simulink model "Control_hibrido"  (R2018a)
settings: Solver=FixedStepAuto  StartTime=0.0  StopTime=20  FixedStep=1e-3  RelTol=1e-3
PreLoadFcn:
  | ej_3_init;
InitFcn:
  | ej_3_init;
StartFcn:
  | hold on;
  | patch([2 0 0 2],[0 2 2 0], [-2 -2 1 1],'g' );
undefined symbols (not defined in the file or in its folder): cfg
libraries: simulink x4, roblocks x2
CloseFcn:
  | hold off;
settings Model: Creator=Guido L  LastModifiedBy=Guido L

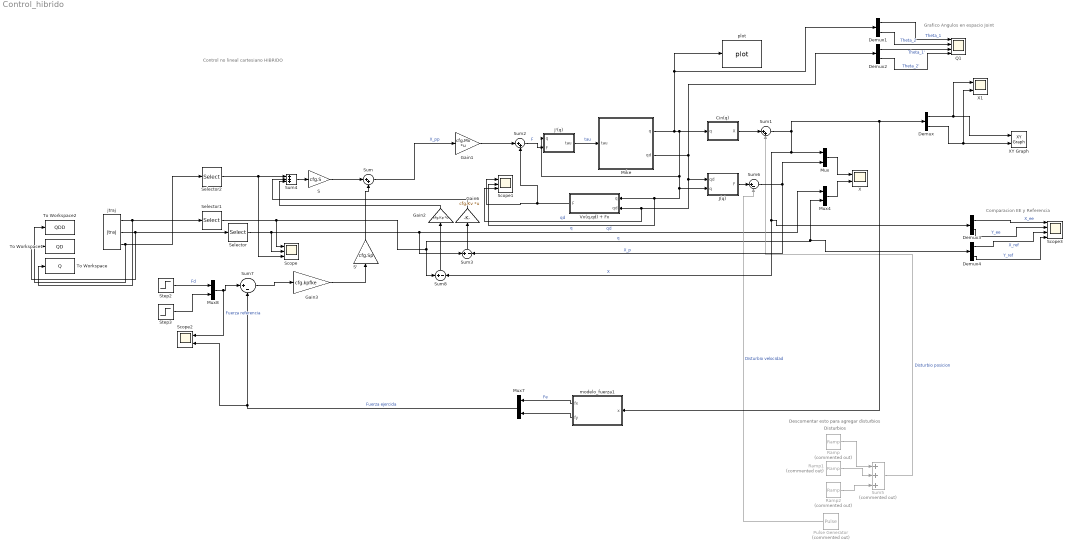
== system Control_hibrido ==
  note: Descomentar esto para agregar disturbios
  note: Control no lineal cartesiano HIBRIDO
  note: Grafico Angulos en espacio Joint
  note: Comparacion EE y Referencia
  note: Disturbios
  Cin(q) : Subsystem
  Demux{,1..4} (5 alike) : Demux  Outputs=2
  Gain1 : Gain  Gain=cfg.Mx  Multiplication=Matrix(K*u) (u vector)
  Gain2 : Gain  Gain=cfg.Kp  Multiplication=Matrix(K*u) (u vector)
  Gain3 : Gain  Gain=cfg.kpfke
  Gain6 : Gain  Gain=cfg.Kv  Multiplication=Matrix(K*u) (u vector)
  J'(q) : Subsystem
  J(q) : Subsystem
  Mike : Subsystem
      mask Display: image('C:\Users\Guido L\Desktop\COntrol\mike_wazowski.jpg');
  Mux{,4,7..8} (4 alike) : Mux  Inputs=2
  Pulse Generator : DiscretePulseGenerator  Commented=on  PulseType=Time based  Period=100  PhaseDelay=5
  Q1 : Scope  NumInputPorts=4
      settings: Tag=qwe
  Ramp : simulink/Sources/Ramp  Commented=on  slope=1  start=5  InitialOutput=0
  Ramp1 : simulink/Sources/Ramp  Commented=on  slope=-2  start=6  InitialOutput=0
  Ramp2 : simulink/Sources/Ramp  Commented=on  slope=1  start=7  InitialOutput=0
  S : Gain  Gain=cfg.S
  S' : Gain  Gain=cfg.Sp
  Scope : Scope  NumInputPorts=3
  Scope1 : Scope  NumInputPorts=3
  Scope2 : Scope  NumInputPorts=2
  Scope3 : Scope  NumInputPorts=4
  Selector : Selector  InputPortWidth=6  IndexOptions=Index vector (dialog)  Indices=[1 2]  OutputSizes=1
  Selector1 : Selector  InputPortWidth=6  IndexOptions=Index vector (dialog)  Indices=[1 2]  OutputSizes=1
  Selector2 : Selector  InputPortWidth=6  IndexOptions=Index vector (dialog)  Indices=[1 2]  OutputSizes=1
  Step2 : Step  After=10  SampleTime=0
  Step3 : Step  After=10  SampleTime=0
  Sum : Sum  Inputs=|++
  Sum1 : Sum  Inputs=|++
  Sum2 : Sum  Inputs=|++
  Sum3 : Sum  Inputs=+-
  Sum4 : Sum  Inputs=+++
  Sum5 : Sum  Commented=on  Inputs=+++
  Sum6 : Sum  Inputs=|+-
  Sum7 : Sum  Inputs=|+-
  Sum8 : Sum  Inputs=+-
  To Workspace : ToWorkspace  VariableName=Q  SaveFormat=Timeseries  SampleTime=-1
  To Workspace1 : ToWorkspace  VariableName=QD  SaveFormat=Timeseries  SampleTime=-1
  To Workspace2 : ToWorkspace  VariableName=QDD  SaveFormat=Timeseries  SampleTime=-1
  Vx(q,qd) + Fx : Subsystem
  X : Scope  NumInputPorts=2
  X1 : Scope  NumInputPorts=2
  XY Graph : simulink/Sinks/XY Graph  xmin=-3  xmax=3  ymin=-3  ymax=3  st=-1
  jtraj : roblocks/Toolbox/jtraj  q0=[1 -1 0 0 0 0]  qf=[1 1 0 0 0 0]  tmax=20  ts=1e-3
  modelo_fuerza1 : MATLAB Function  TreatAsAtomicUnit=on
  plot : roblocks/Arm/plot  robot=Marisol  fps=10  holdplot=on
  wires:
  Mux/1 -> X/1
  Gain1/1 -> Sum2/1
  Selector/1 -> Scope/2, Mux4/1, Sum3/1  "qd"
  jtraj/1 -> To Workspace/1, Selector1/1
  jtraj/2 -> To Workspace1/1, Selector/1
  Mike/1(q) -> Demux1/1, plot/1, Cin(q)/1(q), J(q)/2(q), Scope1/2, Vx(q,qd) + Fx/1(q), J'(q)/2(q)  "q"
  jtraj/3 -> To Workspace2/1, Selector2/1
  Demux/2 -> X1/2, XY Graph/2
  Vx(q,qd) + Fx/1(F) -> Sum2/2, Scope1/1
  Cin(q)/1(X) -> Sum1/1
  Demux/1 -> X1/1, XY Graph/1
  Mux4/1 -> X/2
  Sum/1 -> Gain1/1  "X_pp"
  J(q)/1(F) -> Sum6/1
  Mike/2(qd) -> Demux2/1, Scope1/3, Vx(q,qd) + Fx/2(qd), J(q)/1(qd)  "qd"
  Sum2/1 -> J'(q)/1(F)  "F"
  modelo_fuerza1/1(fx) -> Mux7/1  "Fe"
  modelo_fuerza1/2(fy) -> Mux7/2
  Step2/1 -> Mux8/1  "Fd"
  Sum7/1 -> Gain3/1
  Step3/1 -> Mux8/2
  S'/1 -> Sum/2
  S/1 -> Sum/1
  Sum8/1 -> Gain2/1
  Sum3/1 -> Gain6/1
  Sum4/1 -> S/1
  Gain2/1 -> Sum4/3
  Gain6/1 -> Sum4/2
  Selector2/1 -> Scope/3, Sum4/1
  J'(q)/1(tau) -> Mike/1(tau)  "tau"
  Selector1/1 -> Scope/1, Demux4/1, Mux4/2, Sum8/1  "q"
  Gain3/1 -> S'/1
  Mux8/1 -> Scope2/1, Sum7/1  "Fuerza referencia"
  Mux7/1 -> Scope2/2, Sum7/2  "Fuerza ejercida"
  Demux2/1 -> Q1/3  "Theta_1'"
  Demux1/2 -> Q1/2  "Theta_2"
  Demux1/1 -> Q1/1  "Theta_1"
  Demux2/2 -> Q1/4  "Theta_2'"
  Demux3/2 -> Scope3/2  "Y_ee"
  Demux4/2 -> Scope3/4  "Y_ref"
  Demux4/1 -> Scope3/3  "X_ref"
  Demux3/1 -> Scope3/1  "X_ee"
  Sum5/1 -> Sum1/2  "Disturbio posicion"
  Ramp/1 -> Sum5/1
  Ramp1/1 -> Sum5/2
  Ramp2/1 -> Sum5/3
  Pulse Generator/1 -> Sum6/2  "Disturbio velocidad"
  Sum1/1 -> modelo_fuerza1/1(x), Demux/1, Demux3/1, Sum8/2, Mux/1  "X"
  Sum6/1 -> Mux/2, Sum3/2  "X_p"

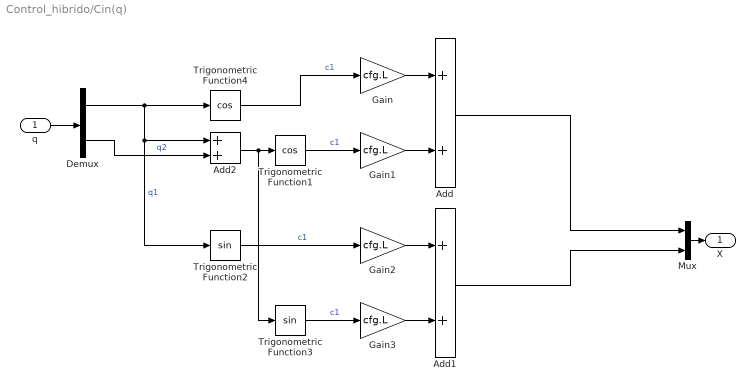
== system Control_hibrido/Cin(q) ==
  q : Inport
  Add : Sum
  Add1 : Sum
  Add2 : Sum
  Demux : Demux  Outputs=2
  Gain{,1..3} (4 alike) : Gain  Gain=cfg.L
  Mux : Mux  Inputs=2
  Trigonometric Function1 : Trigonometry  Operator=cos
  Trigonometric Function2 : Trigonometry
  Trigonometric Function3 : Trigonometry
  Trigonometric Function4 : Trigonometry  Operator=cos
  X : Outport  VectorParamsAs1DForOutWhenUnconnected=on
  wires:
  Demux/1 -> Trigonometric Function2/1, Add2/1, Trigonometric Function4/1  "q1"
  q/1 -> Demux/1
  Mux/1 -> X/1
  Trigonometric Function4/1 -> Gain/1  "c1"
  Gain/1 -> Add/1
  Demux/2 -> Add2/2  "q2"
  Add2/1 -> Trigonometric Function3/1, Trigonometric Function1/1
  Trigonometric Function1/1 -> Gain1/1  "c1"
  Add/1 -> Mux/1
  Gain1/1 -> Add/2
  Trigonometric Function2/1 -> Gain2/1  "c1"
  Gain2/1 -> Add1/1
  Gain3/1 -> Add1/2
  Trigonometric Function3/1 -> Gain3/1  "c1"
  Add1/1 -> Mux/2

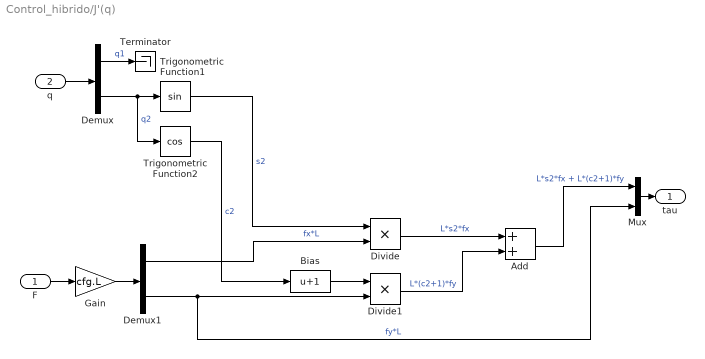
== system Control_hibrido/J'(q) ==
  F : Inport
  q : Inport  Port=2
  Add : Sum
  Bias : Bias  Bias=1
  Demux : Demux  Outputs=2
  Demux1 : Demux  Outputs=2
  Divide : Product  Inputs=**
  Divide1 : Product  Inputs=**
  Gain : Gain  Gain=cfg.L
  Mux : Mux  Inputs=2
  Terminator : Terminator
  Trigonometric Function1 : Trigonometry
  Trigonometric Function2 : Trigonometry  Operator=cos
  tau : Outport  VectorParamsAs1DForOutWhenUnconnected=on
  wires:
  Demux/2 -> Trigonometric Function2/1, Trigonometric Function1/1  "q2"
  Demux/1 -> Terminator/1  "q1"
  q/1 -> Demux/1
  Trigonometric Function1/1 -> Divide/1  "s2"
  Trigonometric Function2/1 -> Bias/1  "c2"
  Demux1/1 -> Divide/2  "fx*L"
  Demux1/2 -> Mux/2, Divide1/2  "fy*L"
  Mux/1 -> tau/1
  F/1 -> Gain/1
  Gain/1 -> Demux1/1
  Divide/1 -> Add/1  "L*s2*fx"
  Bias/1 -> Divide1/1
  Divide1/1 -> Add/2  "L*(c2+1)*fy"
  Add/1 -> Mux/1  "L*s2*fx + L*(c2+1)*fy"

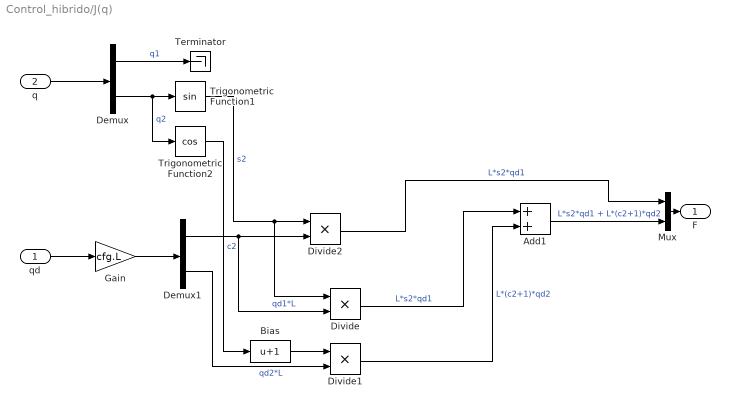
== system Control_hibrido/J(q) ==
  qd : Inport
  q : Inport  Port=2
  Add1 : Sum
  Bias : Bias  Bias=1
  Demux : Demux  Outputs=2
  Demux1 : Demux  Outputs=2
  Divide : Product  Inputs=**
  Divide1 : Product  Inputs=**
  Divide2 : Product  Inputs=**
  Gain : Gain  Gain=cfg.L
  Mux : Mux  Inputs=2
  Terminator : Terminator
  Trigonometric Function1 : Trigonometry
  Trigonometric Function2 : Trigonometry  Operator=cos
  F : Outport  VectorParamsAs1DForOutWhenUnconnected=on
  wires:
  Divide1/1 -> Add1/2  "L*(c2+1)*qd2"
  Divide/1 -> Add1/1  "L*s2*qd1"
  q/1 -> Demux/1
  Bias/1 -> Divide1/1
  Demux/2 -> Trigonometric Function2/1, Trigonometric Function1/1  "q2"
  Gain/1 -> Demux1/1
  Mux/1 -> F/1
  Demux/1 -> Terminator/1  "q1"
  qd/1 -> Gain/1
  Add1/1 -> Mux/2  "L*s2*qd1 + L*(c2+1)*qd2"
  Demux1/1 -> Divide/2, Divide2/2  "qd1*L"
  Trigonometric Function1/1 -> Divide/1, Divide2/1  "s2"
  Divide2/1 -> Mux/1  "L*s2*qd1"
  Demux1/2 -> Divide1/2  "qd2*L"
  Trigonometric Function2/1 -> Bias/1  "c2"

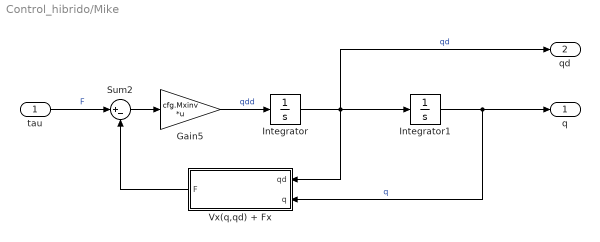
== system Control_hibrido/Mike ==
  tau : Inport
  Gain5 : Gain  Gain=cfg.Mxinv  Multiplication=Matrix(K*u) (u vector)
  Integrator : Integrator  InitialCondition=[0 0]
  Integrator1 : Integrator  InitialCondition=[ -pi/2 pi/2]
  Sum2 : Sum  Inputs=|+-
  Vx(q,qd) + Fx : Subsystem
  q : Outport  VectorParamsAs1DForOutWhenUnconnected=on
  qd : Outport  Port=2  VectorParamsAs1DForOutWhenUnconnected=on
  wires:
  Gain5/1 -> Integrator/1  "qdd"
  Integrator/1 -> Vx(q,qd) + Fx/1(qd), Integrator1/1, qd/1  "qd"
  tau/1 -> Sum2/1  "F"
  Sum2/1 -> Gain5/1
  Integrator1/1 -> Vx(q,qd) + Fx/2(q), q/1  "q"
  Vx(q,qd) + Fx/1(F) -> Sum2/2

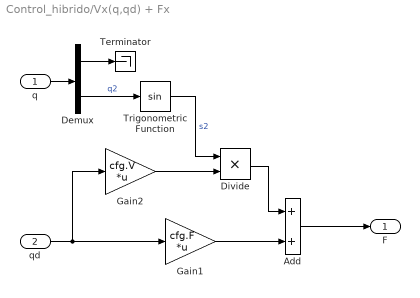
== system Control_hibrido/Vx(q,qd) + Fx ==
  q : Inport
  qd : Inport  Port=2
  Add : Sum
  Demux : Demux  Outputs=2
  Divide : Product  Inputs=**
  Gain1 : Gain  Gain=cfg.F  Multiplication=Matrix(K*u) (u vector)
  Gain2 : Gain  Gain=cfg.V  Multiplication=Matrix(K*u) (u vector)
  Terminator : Terminator
  Trigonometric Function : Trigonometry
  F : Outport  VectorParamsAs1DForOutWhenUnconnected=on
  wires:
  qd/1 -> Gain1/1, Gain2/1
  Gain1/1 -> Add/2
  Add/1 -> F/1
  Gain2/1 -> Divide/2
  q/1 -> Demux/1
  Demux/1 -> Terminator/1
  Demux/2 -> Trigonometric Function/1  "q2"
  Divide/1 -> Add/1
  Trigonometric Function/1 -> Divide/1  "s2"

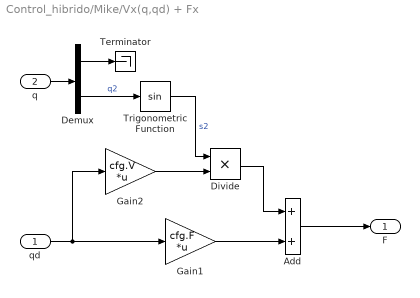
== system Control_hibrido/Mike/Vx(q,qd) + Fx ==
  qd : Inport
  q : Inport  Port=2
  Add : Sum
  Demux : Demux  Outputs=2
  Divide : Product  Inputs=**
  Gain1 : Gain  Gain=cfg.F  Multiplication=Matrix(K*u) (u vector)
  Gain2 : Gain  Gain=cfg.V  Multiplication=Matrix(K*u) (u vector)
  Terminator : Terminator
  Trigonometric Function : Trigonometry
  F : Outport  VectorParamsAs1DForOutWhenUnconnected=on
  wires:
  qd/1 -> Gain1/1, Gain2/1
  Gain1/1 -> Add/2
  Add/1 -> F/1
  Gain2/1 -> Divide/2
  q/1 -> Demux/1
  Demux/1 -> Terminator/1
  Demux/2 -> Trigonometric Function/1  "q2"
  Divide/1 -> Add/1
  Trigonometric Function/1 -> Divide/1  "s2"

== matlab function Control_hibrido/modelo_fuerza1 ==
  data: x input; fx output; fy output
function [fx, fy] = modelo_fuerza(x)
    %La idea es que esto devuelva la reaccion que tiene la pared sobre el
    %end efector cuando este le aplica presión por lo tanto hasta que no
    %choque con la misma no devolvera ningun valor de fuerza
    
wall.m=-1;%pendiente de la funcion que describe la pared
wall.b=2;%ordenada a origen de la misma
wall.ke=1000;%coeficiente de rigidez del cuerpo rigido, del modelo f=ke*x

     x_ee=x(1);
     y_ee=x(2);
     y_pared=wall.m*x_ee+wall.b;
     x_pared= (y_ee-wall.b)/wall.m;
     if((y_ee < y_pared )&&(x_ee < x_pared))%Si no me choque con la pared no hago fuerza
         f=0;
     else
     dist = abs(wall.m*x_ee+2-y_ee)/sqrt(wall.m^2+1); %esto describe la distancia entre la posicion
%     del end efector y la pared por el camino mas corto (Linea ortogonal a la superficie de la pared)
     f=wall.ke*dist;%calculo de la fuerza segun el modelo de rigidez
     end
     fx= f/sqrt(2);
     fy = fx;         

end
